simulink model "MCP_Model_macro_complete"  (R2020a)
settings: configuration reference "globalConfig" (kept outside this file)
InitFcn:
  | load pot.mat;
  | load rpm.mat;
undefined symbols (not defined in the file): pot_kw, rpm, sigbuilder_block
libraries: cstblocks x1
settings Model: OrderedModelArguments=off  Creator=victo  LastModifiedBy=Victor Hugo
settings ConfigSetRef: SourceName=globalConfig  SourceLocation=Base Workspace

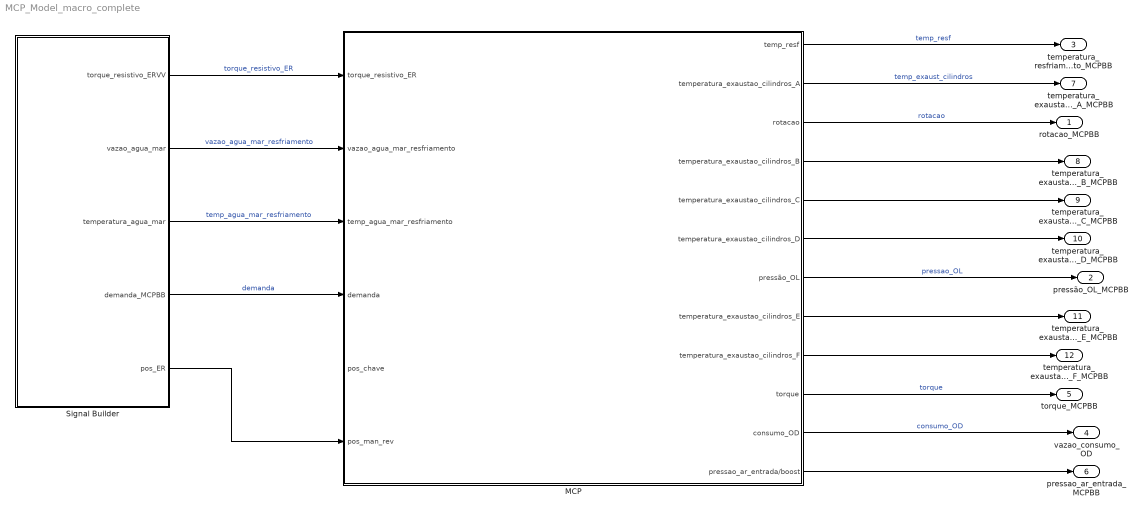
== system MCP_Model_macro_complete ==
  MCP : Subsystem
  Signal Builder : Subsystem  Tag=STV Subsys  LoadFcn=sigbuilder_block('load');  StartFcn=sigbuilder_block('start');  StopFcn=sigbuilder_block('stop');  ClipboardFcn=sigbuilder_block('clipboard');  mask(Sigbuilder block){tuvar=[0:10]}
      mask help: Simulink:masks:SigbuilderBlock_MD
      mask init:
      | if ~strcmp(get_param(bdroot(gcbh),'SimulationStatus'),'stopped') tuvar = sigbuilder_block('maskInit'); end
      settings: CopyFcn=sigbuilder_block('copy');  DeleteFcn=sigbuilder_block('delete');  ModelCloseFcn=sigbuilder_block('modelClose');  PreSaveFcn=sigbuilder_block('preSave');  PauseFcn=sigbuilder_block('pause');  ContinueFcn=sigbuilder_block('continue');  NameChangeFcn=sigbuilder_block('namechange');  OpenFcn=sigbuilder_block('open',[6 30.75 1012.5 447.75 ]);  CloseFcn=sigbuilder_block('close');
      mask Display: plot(0, 0, 100, 100,[2, 2, 32, 32, 2], [68, 8, 8, 68, 68],[32, 2], [38, 38], [32, 19, 2],[53, 60, 44], [32, 17, 17, 2],[16, 16, 31, 31]);txt = getActiveGroup(gcbh);text(2, 100, txt,'verticalAlignment', 'top');
  rotacao_MCPBB : Outport  SignalName=MCPBB0.17
  pressão_OL_MCPBB : Outport  Port=2  SignalName=MCPBB0.18
  temperatura_resfriamento_MCPBB : Outport  Port=3  SignalName=MCPBB0.19
  vazao_consumo_OD : Outport  Port=4  SignalName=MCPBB1.6
  torque_MCPBB : Outport  Port=5  SignalName=MCPBB1.3
  pressao_ar_entrada_MCPBB : Outport  Port=6  SignalName=MCPBB0.20
  temperatura_exaustao_cilindros_A_MCPBB : Outport  Port=7  SignalName=MCPBB0.21
  temperatura_exaustao_cilindros_B_MCPBB : Outport  Port=8  SignalName=MCPBB0.22
  temperatura_exaustao_cilindros_C_MCPBB : Outport  Port=9  SignalName=MCPBB0.23
  temperatura_exaustao_cilindros_D_MCPBB : Outport  Port=10  SignalName=MCPBB0.24
  temperatura_exaustao_cilindros_E_MCPBB : Outport  Port=11  SignalName=MCPBB0.25
  temperatura_exaustao_cilindros_F_MCPBB : Outport  Port=12  SignalName=MCPBB0.26
  wires:
  MCP/1(temp_resf) -> temperatura_resfriamento_MCPBB/1  "temp_resf"
  MCP/2(temperatura_exaustao_cilindros_A) -> temperatura_exaustao_cilindros_A_MCPBB/1  "temp_exaust_cilindros"
  MCP/3(rotacao) -> rotacao_MCPBB/1  "rotacao"
  MCP/4(temperatura_exaustao_cilindros_B) -> temperatura_exaustao_cilindros_B_MCPBB/1
  MCP/5(temperatura_exaustao_cilindros_C) -> temperatura_exaustao_cilindros_C_MCPBB/1
  MCP/6(temperatura_exaustao_cilindros_D) -> temperatura_exaustao_cilindros_D_MCPBB/1
  MCP/7(pressão_OL) -> pressão_OL_MCPBB/1  "pressao_OL"
  MCP/8(temperatura_exaustao_cilindros_E) -> temperatura_exaustao_cilindros_E_MCPBB/1
  MCP/9(temperatura_exaustao_cilindros_F) -> temperatura_exaustao_cilindros_F_MCPBB/1
  MCP/10(torque) -> torque_MCPBB/1  "torque"
  MCP/11(consumo_OD) -> vazao_consumo_OD/1  "consumo_OD"
  MCP/12(pressao_ar_entrada/boost) -> pressao_ar_entrada_MCPBB/1
  Signal Builder/1(torque_resistivo_ERVV) -> MCP/1(torque_resistivo_ER)  "torque_resistivo_ER"
  Signal Builder/2(vazao_agua_mar) -> MCP/2(vazao_agua_mar_resfriamento)  "vazao_agua_mar_resfriamento"
  Signal Builder/3(temperatura_agua_mar) -> MCP/3(temp_agua_mar_resfriamento)  "temp_agua_mar_resfriamento"
  Signal Builder/4(demanda_MCPBB) -> MCP/4(demanda)  "demanda"
  Signal Builder/5(pos_ER) -> MCP/6(pos_man_rev)

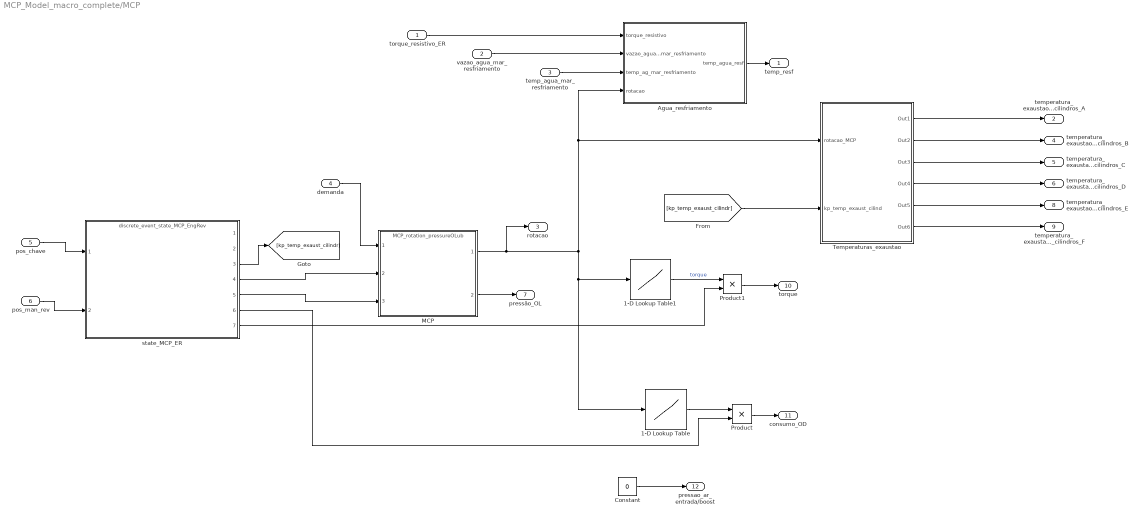
== system MCP_Model_macro_complete/MCP ==
  torque_resistivo_ER : Inport
  vazao_agua_mar_resfriamento : Inport  Port=2
  temp_agua_mar_resfriamento : Inport  Port=3
  demanda : Inport  Port=4
  pos_chave : Inport  Port=5
  pos_man_rev : Inport  Port=6
  1-D Lookup Table : Lookup_n-D  NumberOfTableDimensions=1  BreakpointsForDimension1=[1000,1100,1200,1300,1400,1500,1600,1700,1800,1900]  Table=[25,30,37,45,55,68,82,101,122,145]  InternalRulePriority=Speed  RndMeth=Simplest  InputSameDT=on
  1-D Lookup Table1 : Lookup_n-D  NumberOfTableDimensions=1  BreakpointsForDimension1=rpm  Table=pot_kw./rpm  InternalRulePriority=Speed  RndMeth=Simplest  InputSameDT=on
  Agua_resfriamento : Subsystem  mask{rotacao_nominal_MCP=2000, temp_ambiente=25, temp_max_ag_resf_MCP=90, tal=50}
  Constant : Constant  Value=0
  MCP : ModelReference  ModelNameDialog=MCP_rotation_pressureOLub  SimulationMode=Normal  ModelReferenceVersion=2.8
  Product : Product
  Product1 : Product
  Temperaturas_exaustao : Subsystem
      settings: AttributesFormatString=%<Description>Utilizar relatorio IPqM-REL-156
  state_MCP_ER : ModelReference  ModelNameDialog=discrete_event_state_MCP_EngRev  SimulationMode=Normal  ModelReferenceVersion=2.9
  temp_resf : Outport
  temperatura_exaustao_cilindros_A : Outport  Port=2
  rotacao : Outport  Port=3
  temperatura_exaustao_cilindros_B : Outport  Port=4
  temperatura_exaustao_cilindros_C : Outport  Port=5
  temperatura_exaustao_cilindros_D : Outport  Port=6
  pressão_OL : Outport  Port=7
  temperatura_exaustao_cilindros_E : Outport  Port=8
  temperatura_exaustao_cilindros_F : Outport  Port=9
  torque : Outport  Port=10
  consumo_OD : Outport  Port=11
  pressao_ar_entrada/boost : Outport  Port=12
  wires:
  Constant/1 -> pressao_ar_entrada/boost/1
  Temperaturas_exaustao/5(Out5) -> temperatura_exaustao_cilindros_E/1
  demanda/1 -> MCP/1
  MCP/1 -> 1-D Lookup Table/1, 1-D Lookup Table1/1, Agua_resfriamento/4(rotacao), Temperaturas_exaustao/1(rotacao_MCP), rotacao/1
  Temperaturas_exaustao/1(Out1) -> temperatura_exaustao_cilindros_A/1
  Temperaturas_exaustao/6(Out6) -> temperatura_exaustao_cilindros_F/1
  Temperaturas_exaustao/4(Out4) -> temperatura_exaustao_cilindros_D/1
  Agua_resfriamento/1(temp_agua_resf) -> temp_resf/1
  Temperaturas_exaustao/2(Out2) -> temperatura_exaustao_cilindros_B/1
  temp_agua_mar_resfriamento/1 -> Agua_resfriamento/3(temp_ag_mar_resfriamento)
  Temperaturas_exaustao/3(Out3) -> temperatura_exaustao_cilindros_C/1
  torque_resistivo_ER/1 -> Agua_resfriamento/1(torque_resistivo)
  vazao_agua_mar_resfriamento/1 -> Agua_resfriamento/2(vazao_agua_mar_resfriamento)
  pos_chave/1 -> state_MCP_ER/1
  pos_man_rev/1 -> state_MCP_ER/2
  MCP/2 -> pressão_OL/1
  state_MCP_ER/3 -> [kp_temp_exaust_cilindr]
  state_MCP_ER/4 -> MCP/2
  state_MCP_ER/5 -> MCP/3
  [kp_temp_exaust_cilindr] -> Temperaturas_exaustao/2(kp_temp_exaust_cilind)
  1-D Lookup Table/1 -> Product/1
  Product/1 -> consumo_OD/1
  state_MCP_ER/6 -> Product/2
  1-D Lookup Table1/1 -> Product1/1  "torque"
  Product1/1 -> torque/1
  state_MCP_ER/7 -> Product1/2

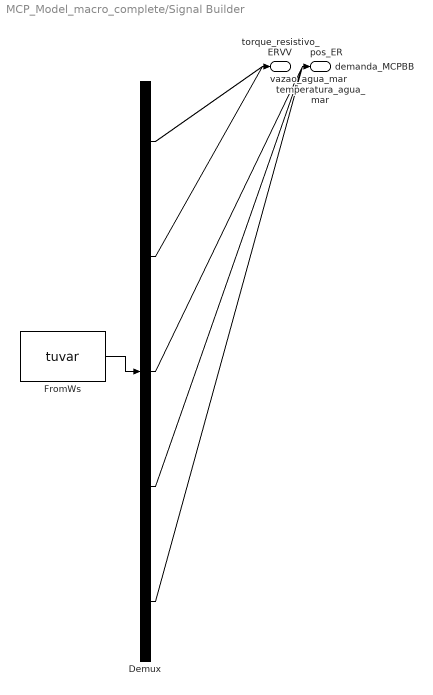
== system MCP_Model_macro_complete/Signal Builder ==
  Demux : Demux  Tag=STV Demux  Outputs=5
      settings: DisplayOption=none
  FromWs : FromWorkspace  Tag=STV FromWs  VariableName=tuvar
      SigBuilderData=|
      | common.afterFinalStr = 'Extrapolate'
      | common.sampleTime = 0
      | dataSet.timeRange = [0 30]
      | dataSet.name = 'Group 1'
      | sbobj.Groups.Name = 'Group 1'
      | sbobj.Groups.Signals(1).Name = 'torque_resistivo_ERVV'
      | sbobj.Groups.Signals(1).XData = [0 2.24 5.06 6 30]
      | sbobj.Groups.Signals(1).YData = [0 0 0 0 0]
      | sbobj.Groups.Signals(2).Name = 'vazao_agua_mar'
      | sbobj.Groups.Signals(2).XData = [0 5 30]
      | sbobj.Groups.Signals(2).YData = [1 1 1]
      | sbobj.Groups.Signals(3).Name = 'temperatura_agua_mar'
      | sbobj.Groups.Signals(3).XData = [0 30]
      | sbobj.Groups.Signals(3).YData = [25 25]
      | sbobj.Groups.Signals(4).Name = 'demanda_MCPBB'
      | sbobj.Groups.Signals(4).XData = [0 1 1 15 15 30]
      | sbobj.Groups.Signals(4).YData = [0 0 800 800 1500 1500]
      | sbobj.Groups.Signals(5).Name = 'pos_ER'
      | sbobj.Groups.Signals(5).XData = [0 10 10 25.05 25.05 30]
      | sbobj.Groups.Signals(5).YData = [0 0 1 1 0 0]
      | sbobj.Groups.TimeRange = [0 30]
  torque_resistivo_ERVV : Outport  Tag=STV Outport
  vazao_agua_mar : Outport  Tag=STV Outport  Port=2
  temperatura_agua_mar : Outport  Tag=STV Outport  Port=3
  demanda_MCPBB : Outport  Tag=STV Outport  Port=4
  pos_ER : Outport  Tag=STV Outport  Port=5
  wires:
  FromWs/1 -> Demux/1
  Demux/1 -> torque_resistivo_ERVV/1
  Demux/2 -> vazao_agua_mar/1
  Demux/3 -> temperatura_agua_mar/1
  Demux/4 -> demanda_MCPBB/1
  Demux/5 -> pos_ER/1

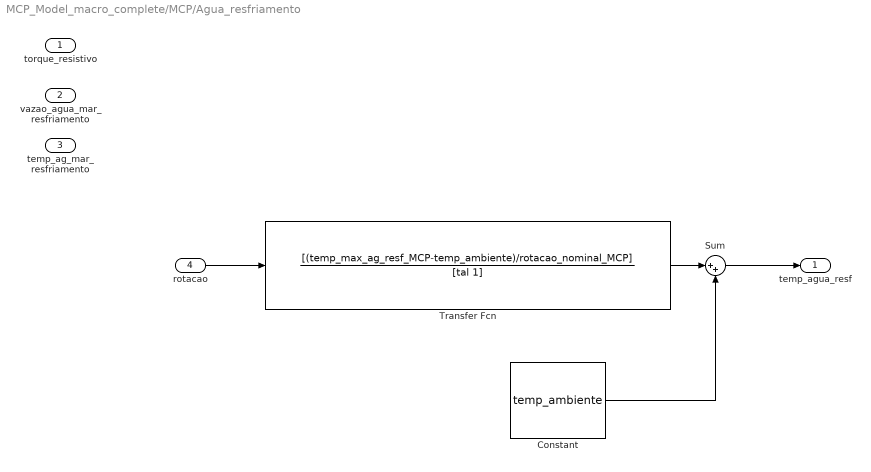
== system MCP_Model_macro_complete/MCP/Agua_resfriamento ==
  torque_resistivo : Inport
  vazao_agua_mar_resfriamento : Inport  Port=2
  temp_ag_mar_resfriamento : Inport  Port=3
  rotacao : Inport  Port=4
  Constant : Constant  Value=temp_ambiente
  Sum : Sum  Inputs=|++
  Transfer Fcn : TransferFcn  Numerator=[(temp_max_ag_resf_MCP-temp_ambiente)/rotacao_nominal_MCP]  Denominator=[tal 1]
  temp_agua_resf : Outport
  wires:
  Constant/1 -> Sum/2
  Sum/1 -> temp_agua_resf/1
  Transfer Fcn/1 -> Sum/1
  rotacao/1 -> Transfer Fcn/1

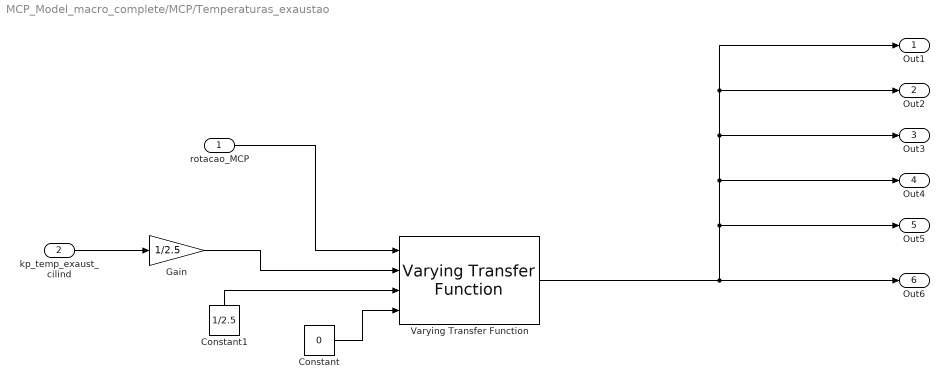
== system MCP_Model_macro_complete/MCP/Temperaturas_exaustao ==
  rotacao_MCP : Inport
  kp_temp_exaust_cilind : Inport  Port=2
  Constant : Constant  Value=0
  Constant1 : Constant  Value=1/2.5
  Gain : Gain  Gain=1/2.5
  Varying Transfer Function : cstblocks/Linear Parameter Varying/Varying Transfer Function  N=1
  Out1 : Outport
  Out2 : Outport  Port=2
  Out3 : Outport  Port=3
  Out4 : Outport  Port=4
  Out5 : Outport  Port=5
  Out6 : Outport  Port=6
  wires:
  rotacao_MCP/1 -> Varying Transfer Function/1
  Varying Transfer Function/1 -> Out3/1, Out2/1, Out1/1, Out4/1, Out5/1, Out6/1
  kp_temp_exaust_cilind/1 -> Gain/1
  Constant/1 -> Varying Transfer Function/4
  Constant1/1 -> Varying Transfer Function/3
  Gain/1 -> Varying Transfer Function/2
